simulink model "DS_distrIntp_4_0_realaxes"  (R2019b)
settings: Solver=FixedStepDiscrete  StartTime=0.0  StopTime=inf  FixedStep=Ts  RelTol=1e-3
StartFcn:
  | close all;
model workspace (MAT data in the model file):
  MvmtPerfEval_collectVal : Simulink.Parameter (value not decoded)
  MvmtPerfEval_sendOwnVal : Simulink.Parameter (value not decoded)
  PAR_center_c2 : Simulink.Parameter (value not decoded)
  PAR_numStepsAheadSmoothing : Simulink.Parameter (value not decoded)
  PAR_startPosReachedTol : Simulink.Parameter (value not decoded)
  PAR_workspace_c2 : Simulink.Parameter (value not decoded)
  PerfEval_numTicks_enable : Simulink.Parameter (value not decoded)
  Segmentregler_I_Gain : Simulink.Parameter (value not decoded)
  Segmentregler_P_Gain : Simulink.Parameter (value not decoded)
  Segmentregler_minVel_enable : Simulink.Parameter (value not decoded)
  Segmentregler_numTicks_enable : Simulink.Parameter (value not decoded)
  Ts : Simulink.Parameter (value not decoded)
  horizon : Simulink.Parameter (value not decoded)
  maxPos_x : Simulink.Parameter (value not decoded)
  maxPos_y : Simulink.Parameter (value not decoded)
  maxPos_z : Simulink.Parameter (value not decoded)
  maxVectorLengths : Simulink.Parameter (value not decoded)
  minAllowedVelSaturation : Simulink.Parameter (value not decoded)
  numAxes : Simulink.Parameter (value not decoded)
  window_length : Simulink.Parameter (value not decoded)
symbols that are objects in the model workspace (value not decoded): MvmtPerfEval_collectVal, MvmtPerfEval_sendOwnVal, numAxes, PAR_center_c2, PAR_numStepsAheadSmoothing, PAR_startPosReachedTol, PAR_workspace_c2, Ts
undefined symbols (not defined in the file or in its folder): DiscIntNeverNeededParam, setP_mat, VelOverride
libraries: vrlib x1, sldrtlib x1
(part 2 of 4)

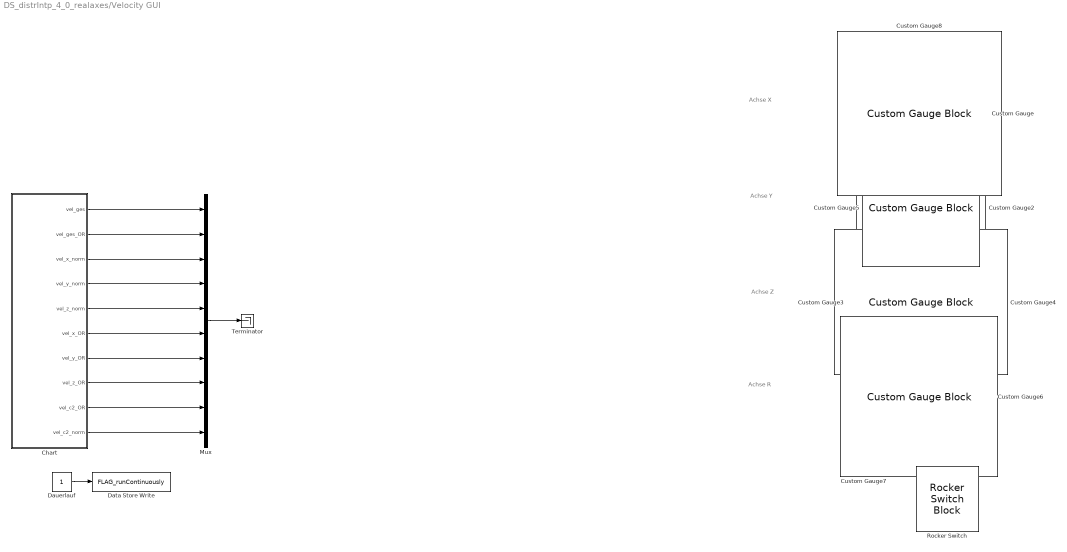
== system DS_distrIntp_4_0_realaxes/Velocity GUI ==
  note: Achse X
  note: Achse Y
  note: Achse Z
  note: Achse R
  Chart : Stateflow chart  BlockKeywords=__PRM__SERIALIZED__DATA__:Stateflow Chart,Stateflow Diagram  TreatAsAtomicUnit=on
  Custom Gauge : CustomGaugeBlock  LabelPosition=Hide  NeedleXPos=0.44289564663671077  NeedleYPos=0.44289564663671077  NeedleHeight=0.14129666921942072  NeedleWidth=0.153010382729839  GaugeArcDefined=true  GaugeArcRadius=0.1662995168673939  GaugeArcStrokeWidth=0.04863239825634951  GaugeArcRotation=240.5385250290321  GaugeArcRatio=0.8333333333333  GaugeArcTransparency=0  ValueArcColor=#1759b0  GaugeTickColor=#000000  ScaleColorsJSON=[]  IsLinearGauge=false  GaugeTrackLeft=0.35  GaugeTrackTop=0.35  GaugeTrackHeight=0.1  GaugeTrackWidth=0.3  GaugeTrackRotation=0
  Custom Gauge2 : CustomGaugeBlock  LabelPosition=Hide  NeedleXPos=0.4446463267949667  NeedleYPos=0.4446463267949667  NeedleHeight=0.1383841830125833  NeedleWidth=0.1383841830125833  GaugeArcDefined=true  GaugeArcRadius=0.15040301426939529  GaugeArcStrokeWidth=0.043983647256998035  GaugeArcRotation=240.5385250290321  GaugeArcRatio=0.8333333333333  GaugeArcTransparency=0  ValueArcColor=#1759b0  GaugeTickColor=#000000  ScaleColorsJSON=[]  IsLinearGauge=false  GaugeTrackLeft=0.35  GaugeTrackTop=0.35  GaugeTrackHeight=0.1  GaugeTrackWidth=0.3  GaugeTrackRotation=0
  Custom Gauge3 : CustomGaugeBlock  LabelPosition=Hide  NeedleImage=data:image/svg+xml;base64,PD94bWwgdmVyc2lvbj0iMS4wIiBlbmNvZGluZz0idXRmLTgiPz4KPCEtLSBHZW5lcmF0b3I6IEFkb2JlIElsbHVzdHJhdG9yIDE5LjIuMSwgU1ZHIEV4cG9ydCBQbHVnLUluIC4gU1ZHIFZlcnNpb246IDYuMDAgQnVpbGQgMCkgIC0tPgo8c3ZnIHZlcnNpb249IjEuMSIgeG1sbnM9Imh0dHA6Ly93d3cudzMub3JnLzIwMDAvc3ZnIiB4bWxuczp4bGluaz0iaHR0cDovL3d3dy53My5vcmcvMTk5OS94bGluayIgeD0iMHB4IiB5PSIwcHgiCgkgdmlld0JveD0iMCAwIDIwMCA1MCIgc3R5bGU9ImVuYWJsZS1iYWNrZ3JvdW5kOm5ldyAw ...(+9940 chars)  NeedleXPos=0.3874876254253927  NeedleYPos=0.4823139286049944  NeedleHeight=0.10899087462396043  NeedleWidth=0.17955441784859344  NeedleInitialRotation=-59.94322499147643  GaugeArcDefined=true  GaugeArcRadius=0.12762379657187173  GaugeArcStrokeWidth=0.037322124674720125  GaugeArcRotation=240.5385250290321  GaugeArcRatio=0.8333333333333  GaugeArcTransparency=0  ValueArcColor=#1759b0  GaugeTickColor=#000000  ScaleColorsJSON=[]  fixedAspectRatio=on  IsLinearGauge=false  GaugeTrackLeft=0.35  GaugeTrackTop=0.35  GaugeTrackHeight=0.1  GaugeTrackWidth=0.3  GaugeTrackRotation=0
  Custom Gauge4 : CustomGaugeBlock  LabelPosition=Hide  NeedleXPos=0.46561993345993286  NeedleYPos=0.46561993345993286  NeedleHeight=0.0840316358512803  NeedleWidth=0.08791249891524028  GaugeArcDefined=true  GaugeArcRadius=0.09341504075538562  GaugeArcStrokeWidth=0.027318163941339572  GaugeArcRotation=240.5385250290321  GaugeArcRatio=0.8333333333333  GaugeArcTransparency=0  ValueArcColor=#1759b0  GaugeTickColor=#000000  ScaleColorsJSON=[]  IsLinearGauge=false  GaugeTrackLeft=0.35  GaugeTrackTop=0.35  GaugeTrackHeight=0.1  GaugeTrackWidth=0.3  GaugeTrackRotation=0
  Custom Gauge5 : CustomGaugeBlock  LabelPosition=Hide  NeedleImage=data:image/svg+xml;base64,PD94bWwgdmVyc2lvbj0iMS4wIiBlbmNvZGluZz0idXRmLTgiPz4KPCEtLSBHZW5lcmF0b3I6IEFkb2JlIElsbHVzdHJhdG9yIDE5LjIuMSwgU1ZHIEV4cG9ydCBQbHVnLUluIC4gU1ZHIFZlcnNpb246IDYuMDAgQnVpbGQgMCkgIC0tPgo8c3ZnIHZlcnNpb249IjEuMSIgeG1sbnM9Imh0dHA6Ly93d3cudzMub3JnLzIwMDAvc3ZnIiB4bWxuczp4bGluaz0iaHR0cDovL3d3dy53My5vcmcvMTk5OS94bGluayIgeD0iMHB4IiB5PSIwcHgiCgkgdmlld0JveD0iMCAwIDIwMCA1MCIgc3R5bGU9ImVuYWJsZS1iYWNrZ3JvdW5kOm5ldyAw ...(+9940 chars)  NeedleXPos=0.3487773586400505  NeedleYPos=0.4762289753305322  NeedleHeight=0.14648955732275654  NeedleWidth=0.24133072862049787  NeedleInitialRotation=-59.94322499147643  GaugeArcDefined=true  GaugeArcRadius=0.171533199712052  GaugeArcStrokeWidth=0.05016292915170857  GaugeArcRotation=240.5385250290321  GaugeArcRatio=0.8333333333333  GaugeArcTransparency=0  ValueArcTransparency=0  ValueArcColor=#1759b0  GaugeTickColor=#000000  ScaleColorsJSON=[]  fixedAspectRatio=on  IsLinearGauge=false  GaugeTrackLeft=0.35  GaugeTrackTop=0.35  GaugeTrackHeight=0.1  GaugeTrackWidth=0.3  GaugeTrackRotation=0
  Custom Gauge6 : CustomGaugeBlock  LabelPosition=Hide  NeedleXPos=0.45342796658839646  NeedleYPos=0.45342796658839646  NeedleHeight=0.11643008352900881  NeedleWidth=0.17803268034034309  GaugeArcDefined=true  GaugeArcRadius=0.12654217507508128  GaugeArcStrokeWidth=0.037005816796108044  GaugeArcRotation=240.5385250290321  GaugeArcRatio=0.8333333333333  GaugeArcTransparency=0  ValueArcColor=#1759b0  GaugeTickColor=#000000  ScaleColorsJSON=[]  IsLinearGauge=false  GaugeTrackLeft=0.35  GaugeTrackTop=0.35  GaugeTrackHeight=0.1  GaugeTrackWidth=0.3  GaugeTrackRotation=0
  Custom Gauge7 : CustomGaugeBlock  LabelPosition=Hide  NeedleImage=data:image/svg+xml;base64,PD94bWwgdmVyc2lvbj0iMS4wIiBlbmNvZGluZz0idXRmLTgiPz4KPCEtLSBHZW5lcmF0b3I6IEFkb2JlIElsbHVzdHJhdG9yIDE5LjIuMSwgU1ZHIEV4cG9ydCBQbHVnLUluIC4gU1ZHIFZlcnNpb246IDYuMDAgQnVpbGQgMCkgIC0tPgo8c3ZnIHZlcnNpb249IjEuMSIgeG1sbnM9Imh0dHA6Ly93d3cudzMub3JnLzIwMDAvc3ZnIiB4bWxuczp4bGluaz0iaHR0cDovL3d3dy53My5vcmcvMTk5OS94bGluayIgeD0iMHB4IiB5PSIwcHgiCgkgdmlld0JveD0iMCAwIDIwMCA1MCIgc3R5bGU9ImVuYWJsZS1iYWNrZ3JvdW5kOm5ldyAw ...(+9940 chars)  NeedleXPos=0.3953411701096402  NeedleYPos=0.48354844483056164  NeedleHeight=0.10138313629943621  NeedleWidth=0.16702123072887018  NeedleInitialRotation=-59.94322499147643  GaugeArcDefined=true  GaugeArcRadius=0.11871545033049134  GaugeArcStrokeWidth=0.034716980352131874  GaugeArcRotation=240.5385250290321  GaugeArcRatio=0.8333333333333  GaugeArcTransparency=0  ValueArcTransparency=0  ValueArcColor=#1759b0  GaugeTickColor=#000000  ScaleColorsJSON=[]  IsLinearGauge=false  GaugeTrackLeft=0.35  GaugeTrackTop=0.35  GaugeTrackHeight=0.1  GaugeTrackWidth=0.3  GaugeTrackRotation=0
  Custom Gauge8 : CustomGaugeBlock  LabelPosition=Hide  NeedleImage=data:image/svg+xml;base64,PD94bWwgdmVyc2lvbj0iMS4wIiBlbmNvZGluZz0idXRmLTgiPz4KPCEtLSBHZW5lcmF0b3I6IEFkb2JlIElsbHVzdHJhdG9yIDE5LjIuMSwgU1ZHIEV4cG9ydCBQbHVnLUluIC4gU1ZHIFZlcnNpb246IDYuMDAgQnVpbGQgMCkgIC0tPgo8c3ZnIHZlcnNpb249IjEuMSIgeG1sbnM9Imh0dHA6Ly93d3cudzMub3JnLzIwMDAvc3ZnIiB4bWxuczp4bGluaz0iaHR0cDovL3d3dy53My5vcmcvMTk5OS94bGluayIgeD0iMHB4IiB5PSIwcHgiCgkgdmlld0JveD0iMCAwIDIwMCA1MCIgc3R5bGU9ImVuYWJsZS1iYWNrZ3JvdW5kOm5ldyAw ...(+9940 chars)  NeedleXPos=0.3937788057820446  NeedleYPos=0.4833028532932101  NeedleHeight=0.10289660053116816  NeedleWidth=0.16951455129355875  NeedleInitialRotation=-59.94322499147643  GaugeArcDefined=true  GaugeArcRadius=0.120487654213576  GaugeArcStrokeWidth=0.03523524117848376  GaugeArcRotation=240.5385250290321  GaugeArcRatio=0.8333333333333  GaugeArcTransparency=0  ValueArcTransparency=0  ValueArcColor=#1759b0  GaugeTickColor=#000000  ScaleColorsJSON=[]  IsLinearGauge=false  GaugeTrackLeft=0.35  GaugeTrackTop=0.35  GaugeTrackHeight=0.1  GaugeTrackWidth=0.3  GaugeTrackRotation=0
  Data Store Write : DataStoreWrite  DataStoreName=FLAG_runContinuously
  Dauerlauf : Constant
  Mux : Mux  Inputs=10
  Rocker Switch : RockerSwitchBlock  LabelPosition=Hide
      settings: Values={{'Dauerlauf AUS', 'Dauerlauf AN'}, [0 1]}
  Terminator : Terminator
  wires:
  Mux/1 -> Terminator/1
  Chart/1(vel_ges) -> Mux/1
  Chart/2(vel_ges_OR) -> Mux/2
  Chart/3(vel_x_norm) -> Mux/3
  Chart/4(vel_y_norm) -> Mux/4
  Chart/5(vel_z_norm) -> Mux/5
  Chart/6(vel_x_OR) -> Mux/6
  Chart/7(vel_y_OR) -> Mux/7
  Chart/8(vel_z_OR) -> Mux/8
  Dauerlauf/1 -> Data Store Write/1
  Chart/9(vel_c2_OR) -> Mux/9
  Chart/10(vel_c2_norm) -> Mux/10

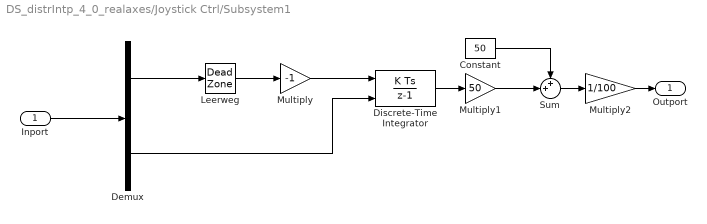
== system DS_distrIntp_4_0_realaxes/Joystick Ctrl/Subsystem1 ==
  Inport : Inport
  Constant : Constant  Value=50
  Demux : Demux  Outputs=2
  Discrete-Time Integrator : DiscreteIntegrator  gainval=0.5  ExternalReset=rising  SampleTime=-1  LimitOutput=on  UpperSaturationLimit=1  LowerSaturationLimit=-0.9  ICPrevOutput=DiscIntNeverNeededParam  ICPrevScaledInput=DiscIntNeverNeededParam
  Leerweg : DeadZone  LowerValue=-0.3  UpperValue=0.3  SaturateOnIntegerOverflow=on
  Multiply : Gain  Gain=-1
  Multiply1 : Gain  Gain=50
  Multiply2 : Gain  Gain=1/100
  Sum : Sum  Inputs=++|
  Outport : Outport  VectorParamsAs1DForOutWhenUnconnected=off
  wires:
  Leerweg/1 -> Multiply/1
  Constant/1 -> Sum/1
  Discrete-Time Integrator/1 -> Multiply1/1
  Multiply/1 -> Discrete-Time Integrator/1
  Multiply1/1 -> Sum/2
  Sum/1 -> Multiply2/1
  Inport/1 -> Demux/1
  Demux/1 -> Leerweg/1
  Demux/2 -> Discrete-Time Integrator/2
  Multiply2/1 -> Outport/1
